simulink model "equalizer"  (R2018b)
settings: Solver=VariableStepAuto  StartTime=0.0  StopTime=307  RelTol=1e-3
libraries: dsparch4 x10, dspmathops x10, dspsnks4 x1, dspvision x1
settings Model: Creator=mrfal  LastModifiedBy=mrfal

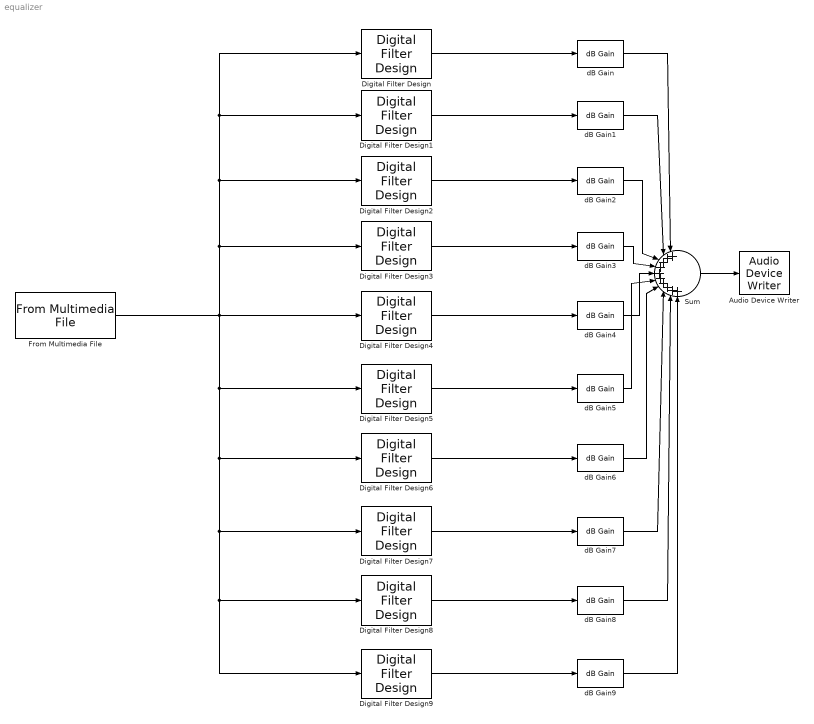
== system equalizer ==
  Audio Device Writer : dspsnks4/Audio Device Writer  Driver=DirectSound  Device=Default  InheritSampleRate=on  SampleRate=44100  BitDepth=16-bit integer  BufferSize=4096  NumBuffers=10  DefaultOutputChannelMapping=on  OutputChannelMapping=1:2  OutputNumUnderrunSamples=off  DriverIdx=1  DeviceWarnFlag=''
  Digital Filter Design{,1..9} (10 alike) : dsparch4/Digital Filter Design  mwdsp_browser_bugfix_var=off
  From Multimedia File : dspvision/From Multimedia File  inputFilename=C:\Users\mrfal\source\repos\Equalizer\The Script - No Good In Goodbye (DriveMusic.me).mp3  loop=on  numPlays=inf  outputStreams=Audio only  videoDataType=single  audioDataType=double  inheritSampleTime=on  userDefinedSampleTime=1/30  noAudioOutput=off  isIntensityVideo=off  fourcc=RGB  colorVideoFormat=Separate color signals  outputEOF=off  dataOrg=Column-major  audioFrameSize=1024  computeAudioFrameSize=off  outSamplingMode=Sample based
      settings: SourceProductBaseCode=VP
  Sum : Sum  Inputs=|++++++++++
  dB Gain{,1..9} (10 alike) : dspmathops/dB Gain  dB=0  intype=Amplitude
      settings: SourceProductName=DSP System Toolbox  SourceProductBaseCode=DS
  wires:
  Digital Filter Design/1 -> dB Gain/1
  Digital Filter Design1/1 -> dB Gain1/1
  Digital Filter Design2/1 -> dB Gain2/1
  Digital Filter Design3/1 -> dB Gain3/1
  Digital Filter Design4/1 -> dB Gain4/1
  Digital Filter Design5/1 -> dB Gain5/1
  Digital Filter Design6/1 -> dB Gain6/1
  Digital Filter Design7/1 -> dB Gain7/1
  Digital Filter Design8/1 -> dB Gain8/1
  Digital Filter Design9/1 -> dB Gain9/1
  Sum/1 -> Audio Device Writer/1
  From Multimedia File/1 -> Digital Filter Design5/1, Digital Filter Design6/1, Digital Filter Design7/1, Digital Filter Design8/1, Digital Filter Design9/1, Digital Filter Design3/1, Digital Filter Design2/1, Digital Filter Design1/1, Digital Filter Design/1, Digital Filter Design4/1
  dB Gain/1 -> Sum/1
  dB Gain1/1 -> Sum/2
  dB Gain2/1 -> Sum/3
  dB Gain3/1 -> Sum/4
  dB Gain4/1 -> Sum/5
  dB Gain5/1 -> Sum/6
  dB Gain6/1 -> Sum/7
  dB Gain7/1 -> Sum/8
  dB Gain8/1 -> Sum/9
  dB Gain9/1 -> Sum/10
